simulink model "Microgrid_No_Attack"  (R2020b)
settings: Solver=VariableStepAuto  StartTime=0.0  StopTime=0.25  RelTol=1e-3
undefined symbols (not defined in the file): A_state_matrix_DG1, A_state_matrix_DG2, A_state_matrix_DG3, A_state_matrix_DG4, B_input_matrix_DG1, B_input_matrix_DG2, B_input_matrix_DG3, B_input_matrix_DG4, C_output_matrix_DG1, C_output_matrix_DG2, C_output_matrix_DG3, C_output_matrix_DG4, L_dot_DG1, L_dot_DG2, L_dot_DG3, L_dot_DG4
(part 2 of 2)

== matlab function Microgrid_No_Attack/vomag ==
  data: x9 input; x10 input; x24 input; vomag_1DG output; x25 input; x39 input; vomag_2DG output; vomag_3DG output; vomag_4DG output; x40 input; x54 input; x55 input
function [vomag_1DG,vomag_2DG,vomag_3DG,vomag_4DG] = vomag(x9,x10,x24,x25,x39,x40,x54,x55)


vomag_1DG= sqrt((x9^2) + (x10^2));
vomag_2DG= sqrt((x24^2) + (x25^2));
vomag_3DG= sqrt((x39^2) + (x40^2));
vomag_4DG= sqrt((x54^2) + (x55^2));

== matlab function Microgrid_No_Attack/NET ==
  data: x53 input; x54 input; x55 input; xdot53 output; xdot54 output; xdot55 output; xdot56 output; x56 input; x57 input; x58 input; vbD1 input; vbQ1 input; vbD2 input; vbQ2 input; vbD3 input; vbQ3 input; vbD4 input; vbQ4 input; xdot57 output; xdot58 output; wcom input
function [xdot53,xdot54,xdot55,xdot56,xdot57,xdot58] = Net(x53,x54,x55,x56,x57,x58,vbD1,vbQ1,vbD2,vbQ2,vbD3,vbQ3,vbD4,vbQ4,wcom)
% This block supports an embeddable subset of the MATLAB language.
% See the help menu for details. 
%%%--------Parameter values--------------
Cf=50e-6;Lf=1.35e-3;rLf=.1;
Lc=.35e-3;rLc=.03;
wc=31.41;
mp1=9.4e-5;mp2=mp1;mp3=12.5e-5;mp4=mp3;


nq1=1.3e-3;nq2=nq1;nq3=1.5e-3;nq4=nq3;


Kpv1=.1;Kiv1=420;Kpv2=Kpv1;Kiv2=Kiv1;
Kpc1=15;Kic1=20*10^3;Kpc2=Kpc1;Kic2=Kic1;


Kpv3=.05;Kiv3=390;Kpv4=Kpv3;Kiv4=Kiv3;
Kpc3=10.5;Kic3=16*10^3;Kpc4=Kpc3;Kic4=Kic3;


F=.75;

% kp=285;tau=0.00002;
%---------------
% rN=1e4;
% wb=2*pi*50;
% wref=2*pi*50;
% 
% Vn=380;
% Vdref=1*Vn;
% Vqref=0;
%-----Network Data-------
rline1=.23;Lline1=318e-6;
rline2=.35;Lline2=1847e-6;
rline3=.23;Lline3=318e-6;

Rload1=30;
Lload1=15/(2*pi*50);
Rload2=20;
Lload2=10/(2*pi*50);
Rload3=25;
Lload3=10/(2*pi*50);
Rload4=25;
Lload4=15/(2*pi*50);

%----1->2-----line1
xdot53=(-rline1/Lline1)*x53+wcom*x54+(1/Lline1)*(vbD1-vbD2); %ilineD1_dot
xdot54=(-rline1/Lline1)*x54-wcom*x53+(1/Lline1)*(vbQ1-vbQ2); %ilineQ1_dot
%----2->3-----line2
xdot55=(-rline2/Lline2)*x55+wcom*x56+(1/Lline2)*(vbD2-vbD3); %ilineD2_dot
xdot56=(-rline2/Lline2)*x56-wcom*x55+(1/Lline2)*(vbQ2-vbQ3); %ilineQ2_dot
%----3->4-----line3
xdot57=(-rline3/Lline3)*x57+wcom*x58+(1/Lline3)*(vbD3-vbD4); %ilineD3_dot
xdot58=(-rline3/Lline3)*x58-wcom*x57+(1/Lline3)*(vbQ3-vbQ4); %ilineQ3_dot

== matlab function Microgrid_No_Attack/LOAD ==
  data: x59 input; x60 input; x61 input; xdot59 output; xdot60 output; xdot61 output; xdot62 output; x62 input; x63 input; x64 input; x65 input; x66 input; vbD1 input; vbQ1 input; vbD2 input; vbQ2 input; vbD3 input; vbQ3 input; vbD4 input; vbQ4 input; wcom input; xdot63 output; xdot64 output; xdot65 output; xdot66 output
function [xdot59,xdot60,xdot61,xdot62,xdot63,xdot64,xdot65,xdot66] = Load(x59,x60,x61,x62,x63,x64,x65,x66,vbD1,vbQ1,vbD2,vbQ2,vbD3,vbQ3,vbD4,vbQ4,wcom)
% This block supports an embeddable subset of the MATLAB language.
% See the help menu for details. 
%%%--------Parameter values--------------
Cf=50e-6;Lf=1.35e-3;rLf=.1;
Lc=.35e-3;rLc=.03;
wc=31.41;
mp1=9.4e-5;mp2=mp1;mp3=12.5e-5;mp4=mp3;


nq1=1.3e-3;nq2=nq1;nq3=1.5e-3;nq4=nq3;


Kpv1=.1;Kiv1=420;Kpv2=Kpv1;Kiv2=Kiv1;
Kpc1=15;Kic1=20*10^3;Kpc2=Kpc1;Kic2=Kic1;


Kpv3=.05;Kiv3=390;Kpv4=Kpv3;Kiv4=Kiv3;
Kpc3=10.5;Kic3=16*10^3;Kpc4=Kpc3;Kic4=Kic3;


F=.75;

% kp=285;tau=0.00002;
%---------------
% rN=1e4;
% wb=2*pi*50;
% wref=2*pi*50;
% 
% Vn=380;
% Vdref=1*Vn;
% Vqref=0;
%-----Network Data-------
rline1=.23;Lline1=318e-6;
rline2=.35;Lline2=1847e-6;
rline3=.23;Lline3=318e-6;
% rline4=.35;Lline4=.58/(2*pi*50);
% rline5=.23;Lline5=.1/(2*pi*50);
% rline6=.35;Lline6=.58/(2*pi*50);
% rline7=.23;Lline7=.1/(2*pi*50);

Rload1=30;
Lload1=15/(2*pi*50);
Rload2=20;
Lload2=10/(2*pi*50);
Rload3=25;
Lload3=10/(2*pi*50);
Rload4=25;
Lload4=15/(2*pi*50);

%------Load1--------
xdot59=(-Rload1/Lload1)*x59+wcom*x60+(1/Lload1)*vbD1; %iloadD1_dot
xdot60=(-Rload1/Lload1)*x60-wcom*x59+(1/Lload1)*vbQ1; %iloadQ1_dot
%------Load2--------
xdot61=(-Rload2/Lload2)*x61+wcom*x62+(1/Lload2)*vbD2; %iloadD2_dot
xdot62=(-Rload2/Lload2)*x62-wcom*x61+(1/Lload2)*vbQ2; %iloadQ2_dot
%------Load3--------
xdot63=(-Rload3/Lload3)*x63+wcom*x64+(1/Lload3)*vbD3; %iloadD3_dot
xdot64=(-Rload3/Lload3)*x64-wcom*x63+(1/Lload3)*vbQ3; %iloadQ3_dot
%------Load4--------
xdot65=(-Rload4/Lload4)*x65+wcom*x66+(1/Lload4)*vbD4; %iloadD4_dot
xdot66=(-Rload4/Lload4)*x66-wcom*x65+(1/Lload4)*vbQ4; %iloadQ4_dot

== matlab function Microgrid_No_Attack/omega_1DG ==
  data: x1_1DG input; w1 output; x14_1DG input
function w1  = omega_1DG(x1_1DG,x14_1DG)

mp1=9.4e-5;mp2=mp1;mp3=12.5e-5;mp4=mp3;

w1= x14_1DG -mp1*x1_1DG;

== matlab function Microgrid_No_Attack/VB ==
  data: vbD1 output; vbQ1 output; vbD2 output; vbQ2 output; ilineD1 input; ilineQ1 input; ilineD2 input; vbD3 output; vbQ3 output; ilineQ2 input; ilineD3 input; ilineQ3 input; iloadD1 input; iloadQ1 input; iloadD2 input; iloadQ2 input; iloadD3 input; iloadQ3 input; iloadD4 input; iloadQ4 input; ioD1 input; ioQ1 input; ioD2 input; ioQ2 input; ioD3 input; ioQ3 input; ioD4 input; ioQ4 input; vbD4 output; vbQ4 output
function [vbD1,vbQ1,vbD2,vbQ2,vbD3,vbQ3,vbD4,vbQ4] = VB(ilineD1,ilineQ1,ilineD2,ilineQ2,ilineD3,ilineQ3,iloadD1,iloadQ1,iloadD2,iloadQ2,iloadD3,iloadQ3,iloadD4,iloadQ4,ioD1,ioQ1,ioD2,ioQ2,ioD3,ioQ3,ioD4,ioQ4)
% This block supports an embeddable subset of the MATLAB language.
% See the help menu for details. 
%%%--------Parameter values--------------


vbD1= (ioD1 - ilineD1 - iloadD1); vbQ1= (ioQ1 - ilineQ1 - iloadQ1);
vbD2= (ioD2 + ilineD1 - ilineD2 - iloadD2); vbQ2= (ioQ2 + ilineQ1 - ilineQ2 - iloadQ2);
vbD3= (ioD3 + ilineD2 - ilineD3 - iloadD3); vbQ3= (ioQ3 + ilineQ2 - ilineQ3 - iloadQ3);
vbD4= (ioD4 + ilineD3 - iloadD4); vbQ4= (ioQ4 + ilineQ3 - iloadQ4);

== matlab function Microgrid_No_Attack/omega_2DG ==
  data: x16_2DG input; w2 output; x29_2DG input
function w2  = omega_2DG(x16_2DG,x29_2DG)

mp1=9.4e-5;mp2=mp1;mp3=12.5e-5;mp4=mp3;

w2= x29_2DG -mp2*x16_2DG;

== matlab function Microgrid_No_Attack/omega_3DG ==
  data: x31_3DG input; w3 output; x44_3DG input
function w3  = omega_3DG(x31_3DG,x44_3DG)

mp1=9.4e-5;mp2=mp1;mp3=12.5e-5;mp4=mp3;

w3= x44_3DG -mp3*x31_3DG;

== matlab function Microgrid_No_Attack/Frequencies ==
  data: w1 input; f1 output; w2 input; w3 input; w4 input; f2 output; f3 output; f4 output
function [f1,f2,f3,f4] = frequencies(w1,w2,w3,w4)

f1 = w1/(2*pi);
f2 = w2/(2*pi);
f3 = w3/(2*pi);
f4 = w4/(2*pi);

== matlab function Microgrid_No_Attack/omega_4DG ==
  data: x46_4DG input; w4 output; x59_4DG input
function w4  = omega_4DG(x46_4DG,x59_4DG)

mp1=9.4e-5;mp2=mp1;mp3=12.5e-5;mp4=mp3;

w4= x59_4DG -mp4*x46_4DG;

== matlab function Microgrid_No_Attack/OBSERVER DG 1 ==
  data: A_state_matrix_DG1 input; x_hat_dot_DG1 output size=15; B_input_matrix_DG1 input; C_output_matrix_DG1 input; L_dot_DG1 input; y_DG1 input; u_vector_DG1 input; x1_hat input; x2_hat input; x3_hat input; x4_hat input; x5_hat input; x6_hat input; x7_hat input; x8_hat input; x9_hat input; x10_hat input; x11_hat input; x12_hat input; x13_hat input; x14_hat input; x15_hat input; y_hat_DG1 output size=15
function [x_hat_dot_DG1,y_hat_DG1] = observer_DG1(A_state_matrix_DG1,B_input_matrix_DG1,C_output_matrix_DG1,L_dot_DG1,y_DG1,u_vector_DG1, x1_hat,x2_hat,x3_hat,x4_hat,x5_hat,x6_hat,x7_hat,x8_hat,x9_hat,x10_hat,x11_hat,x12_hat,x13_hat,x14_hat,x15_hat)

Cf=50e-6;Lf=1.35e-3;rLf=.1;
Lc=.35e-3;rLc=.03;
wc=31.41;
mp1=9.4e-5;mp2=mp1;mp3=12.5e-5;mp4=mp3;


nq1=1.3e-3;nq2=nq1;nq3=1.5e-3;nq4=nq3;


Kpv1=.1;Kiv1=420;Kpv2=Kpv1;Kiv2=Kiv1;
Kpc1=15;Kic1=20*10^3;Kpc2=Kpc1;Kic2=Kic1;


Kpv3=.05;Kiv3=390;Kpv4=Kpv3;Kiv4=Kiv3;
Kpc3=10.5;Kic3=16*10^3;Kpc4=Kpc3;Kic4=Kic3;


F=.75;

wb=2*pi*50;

%% Non linear function (f) 15x1 

f_nonlinear_function_hat=[
(wc*x9_hat*x11_hat) + (wc*x10_hat*x12_hat);
(-wc*x9_hat*x12_hat) + (wc*x10_hat*x11_hat);
0;
0;
0;
0;
(x14_hat*x8_hat) - (mp1*x1_hat*x8_hat);
(-x14_hat*x7_hat) + (mp1*x1_hat*x7_hat);
(x14_hat*x10_hat) - (mp1*x1_hat*x10_hat);
(-x14_hat*x9_hat) + (mp1*x1_hat*x9_hat);
(x14_hat*x12_hat) - (mp1*x1_hat*x12_hat);
(-x14_hat*x11_hat) + (mp1*x1_hat*x11_hat);
0;
0;
0;
];

%% L'' hat DG 1

%L'' is 15x15, L' is 15x15, therefore L is 15x15

L_dot_dot_DG1= zeros(15,15)

L_dot_dot_DG1(1,7)= mp1*x8_hat;
L_dot_dot_DG1(1,8)= -mp1*x7_hat;
L_dot_dot_DG1(1,9)= mp1*x10_hat;
L_dot_dot_DG1(1,10)= -mp1*x9_hat;
L_dot_dot_DG1(1,11)= mp1*x12_hat - wc*x9_hat;
L_dot_dot_DG1(1,12)= -mp1*x11_hat - wc*x10_hat;
L_dot_dot_DG1(2,11)= -wc*x10_hat;
L_dot_dot_DG1(2,12)= wc*x9_hat;
L_dot_dot_DG1(7,14)= -x8_hat;
L_dot_dot_DG1(8,14)= x7_hat;
L_dot_dot_DG1(9,14)= -x10_hat;
L_dot_dot_DG1(10,14)= x9_hat;
L_dot_dot_DG1(11,14)= -x12_hat;
L_dot_dot_DG1(12,14)= x11_hat;



%% non linear gain L hat

L_hat_DG1= L_dot_DG1 + L_dot_dot_DG1

%% x hat vector

x_hat_vector_DG1= [x1_hat;x2_hat;x3_hat;x4_hat;x5_hat;x6_hat;x7_hat;x8_hat;x9_hat;x10_hat;x11_hat;x12_hat;x13_hat;x14_hat;x15_hat];
%% x hat dot

y_hat_DG1= C_output_matrix_DG1*x_hat_vector_DG1

x_hat_dot_DG1= A_state_matrix_DG1*x_hat_vector_DG1 + f_nonlinear_function_hat + B_input_matrix_DG1*u_vector_DG1 + L_hat_DG1*(y_DG1 - y_hat_DG1)

== matlab function Microgrid_No_Attack/DG 1 Matrices ==
  data: x1 input; x_dot_DG1 output; x2 input; x3 input; x4 input; x5 input; x6 input; x7 input; x8 input; x9 input; x10 input; x11 input; x12 input; x13 input; x14 input; x15 input; y_DG1 output; P_matrix input; Q_matrix input; w_matrix input; v_od_matrix input; wcom input; vbD1 input; vbQ1 input; A_state_matrix_DG1 input; B_input_matrix_DG1 input; C_output_matrix_DG1 input; ioD1 output; ioQ1 output; u_vector_DG1 output; vbd1 output; vbq1 output
function [x_dot_DG1, y_DG1, ioD1, ioQ1, u_vector_DG1,vbd1,vbq1] = Matrices_SSM_DG1(x1,x2,x3,x4,x5,x6,x7,x8,x9,x10,x11,x12,x13,x14,x15,P_matrix, Q_matrix, w_matrix, v_od_matrix,wcom,vbD1,vbQ1,A_state_matrix_DG1,B_input_matrix_DG1,C_output_matrix_DG1)



Cf=50e-6;Lf=1.35e-3;rLf=.1;
Lc=.35e-3;rLc=.03;
wc=31.41;
mp1=9.4e-5;mp2=mp1;mp3=12.5e-5;mp4=mp3;


nq1=1.3e-3;nq2=nq1;nq3=1.5e-3;nq4=nq3;


Kpv1=.1;Kiv1=420;Kpv2=Kpv1;Kiv2=Kiv1;
Kpc1=15;Kic1=20*10^3;Kpc2=Kpc1;Kic2=Kic1;


Kpv3=.05;Kiv3=390;Kpv4=Kpv3;Kiv4=Kiv3;
Kpc3=10.5;Kic3=16*10^3;Kpc4=Kpc3;Kic4=Kic3;


F=.75;

wb=2*pi*50;

A_matrix= [0 0 0 0; 1 0 0 0; 1 0 0 0; 1 0 0 0]; %associated adjacency matrix
g_pinning_gain= [1;0;0;0]; %pinning gain vector
w_ref= 2*pi*50;
v_ref= 1;
c_f_1DG= 30;
c_v_1DG= 30;

m_P_1DG= 9.4*10^-5;
m_P_2DG= 9.4*10^-5;
m_P_3DG= 12.5*10^-5;
m_P_4DG= 12.5*10^-5;
n_Q_1DG= 1.3*10^-3;
n_Q_2DG= 1.3*10^-3; 
n_Q_3DG= 1.5*10^-3; 
n_Q_4DG= 1.5*10^-3; 

m_P_matrix= [m_P_1DG; m_P_2DG; m_P_3DG; m_P_4DG];
n_Q_matrix= [n_Q_1DG; n_Q_2DG; n_Q_3DG; n_Q_4DG];

vbd1=cos(0)*vbD1+sin(0)*vbQ1;vbq1=-sin(0)*vbD1+cos(0)*vbQ1;

%% Extracting several terms for x dot 14

%Obtaining wj_input (cf*sum_aij*wj)

wj_input= 0;

for i=1
    for j= 1:4
        wj_input= (A_matrix(i,j)*w_matrix(j)) + wj_input;
    end
end

wj_input= wj_input*c_f_1DG;



%Obtaining wref_input (cf*gi*wref)


wref_input= c_f_1DG*g_pinning_gain(i)*w_ref;



%Obtaining Pj_input (cf*sum_aij*Pj)

Pj_input= 0;

for i= 1
    for j= 1:4
        Pj_input= (A_matrix(i,j)*m_P_matrix(j)*P_matrix(j)) + Pj_input;
    end
end

Pj_input= Pj_input*c_f_1DG;


        
%% Extracting several terms for x dot 15


%Obtaining vodj_input (cv*sum_aij*vodj)

vodj_input= 0;

for i= 1
    for j= 1:4
        vodj_input= (A_matrix(i,j)*v_od_matrix(j)) + vodj_input;
    end
end

vodj_input= c_v_1DG*vodj_input;


%Obtaining vref_input (cv*gi*vref)

vref_input= c_v_1DG*g_pinning_gain(i)*v_ref;


%Obtaining Qj_input (cv*sum_aij*Qj)

Qj_input= 0;

for i= 1
    for j= 1:4
        Qj_input= (A_matrix(i,j)*n_Q_matrix(j)*Q_matrix(j)) + Qj_input;
    end
end

Qj_input= c_v_1DG*Qj_input;




%% A matrix calculation

%A has 15 rows 15 columns

% x_vector=[P_i, Q_i, fi_d_i, fi_q_i,gamma_d_i,gamma_q_i, il_d_i, il_q_i, vo_d_i, vo_q_i,io_d_i,io_q_i,alpha_i,wni,Vni];


%% B Matrix Calculation 

%B has 15 rows 9 columns

u_vector_DG1= [wcom;vbd1;vbq1;wj_input;wref_input;Pj_input;vodj_input;vref_input;Qj_input];



%% C matrix calculation

% y=[states from 1 to 15]

%C has 15 rows 15 columns, C equal to identity matrix


%% Non linear function (f) 15x1 

f_nonlinear_function=[
(wc*x9*x11) + (wc*x10*x12);
(-wc*x9*x12) + (wc*x10*x11);
0;
0;
0;
0;
(x14*x8) - (mp1*x1*x8);
(-x14*x7) + (mp1*x1*x7);
(x14*x10) - (mp1*x1*x10);
(-x14*x9) + (mp1*x1*x9);
(x14*x12) - (mp1*x1*x12);
(-x14*x11) + (mp1*x1*x11);
0;
0;
0;
];


%% x vector

x_vector_DG1= [x1;x2;x3;x4;x5;x6;x7;x8;x9;x10;x11;x12;x13;x14;x15];
%% xdot
x_dot_DG1= A_state_matrix_DG1*x_vector_DG1 + f_nonlinear_function + B_input_matrix_DG1*u_vector_DG1

y_DG1= C_output_matrix_DG1*x_vector_DG1



ioD1=cos(0)*x11-sin(0)*x12;
ioQ1=sin(0)*x11+cos(0)*x12;

== matlab function Microgrid_No_Attack/OBSERVER DG 2 ==
  data: A_state_matrix_DG2 input; x_hat_dot_DG2 output; B_input_matrix_DG2 input; C_output_matrix_DG2 input; L_dot_DG2 input; y_DG2 input; u_vector_DG2 input; x1_hat input; x2_hat input; x3_hat input; x4_hat input; x5_hat input; x6_hat input; x7_hat input; x8_hat input; x9_hat input; x10_hat input; x11_hat input; x12_hat input; x13_hat input; x14_hat input; x15_hat input; y_hat_DG2 output
function [x_hat_dot_DG2,y_hat_DG2] = observer_DG2(A_state_matrix_DG2,B_input_matrix_DG2,C_output_matrix_DG2,L_dot_DG2,y_DG2,u_vector_DG2, x1_hat,x2_hat,x3_hat,x4_hat,x5_hat,x6_hat,x7_hat,x8_hat,x9_hat,x10_hat,x11_hat,x12_hat,x13_hat,x14_hat,x15_hat)

Cf=50e-6;Lf=1.35e-3;rLf=.1;
Lc=.35e-3;rLc=.03;
wc=31.41;
mp1=9.4e-5;mp2=mp1;mp3=12.5e-5;mp4=mp3;


nq1=1.3e-3;nq2=nq1;nq3=1.5e-3;nq4=nq3;


Kpv1=.1;Kiv1=420;Kpv2=Kpv1;Kiv2=Kiv1;
Kpc1=15;Kic1=20*10^3;Kpc2=Kpc1;Kic2=Kic1;


Kpv3=.05;Kiv3=390;Kpv4=Kpv3;Kiv4=Kiv3;
Kpc3=10.5;Kic3=16*10^3;Kpc4=Kpc3;Kic4=Kic3;


F=.75;

wb=2*pi*50;

%% Non linear function (f) 15x1 

f_nonlinear_function_hat=[
(wc*x9_hat*x11_hat) + (wc*x10_hat*x12_hat);
(-wc*x9_hat*x12_hat) + (wc*x10_hat*x11_hat);
0;
0;
0;
0;
(x14_hat*x8_hat) - (mp1*x1_hat*x8_hat);
(-x14_hat*x7_hat) + (mp1*x1_hat*x7_hat);
(x14_hat*x10_hat) - (mp1*x1_hat*x10_hat);
(-x14_hat*x9_hat) + (mp1*x1_hat*x9_hat);
(x14_hat*x12_hat) - (mp1*x1_hat*x12_hat);
(-x14_hat*x11_hat) + (mp1*x1_hat*x11_hat);
0;
0;
0;
];

%% L'' hat DG 2

%L'' is 15x15, L' is 15x15, therefore L is 15x15

L_dot_dot_DG2= zeros(15,15)

L_dot_dot_DG2(1,7)= mp2*x8_hat;
L_dot_dot_DG2(1,8)= -mp2*x7_hat;
L_dot_dot_DG2(1,9)= mp2*x10_hat;
L_dot_dot_DG2(1,10)= -mp2*x9_hat;
L_dot_dot_DG2(1,11)= mp2*x12_hat - wc*x9_hat;
L_dot_dot_DG2(1,12)= -mp2*x11_hat - wc*x10_hat;
L_dot_dot_DG2(2,11)= -wc*x10_hat;
L_dot_dot_DG2(2,12)= wc*x9_hat;
L_dot_dot_DG2(7,14)= -x8_hat;
L_dot_dot_DG2(8,14)= x7_hat;
L_dot_dot_DG2(9,14)= -x10_hat;
L_dot_dot_DG2(10,14)= x9_hat;
L_dot_dot_DG2(11,14)= -x12_hat;
L_dot_dot_DG2(12,14)= x11_hat;

%% non linear gain L hat

L_hat_DG2= L_dot_DG2 + L_dot_dot_DG2

%% x hat vector

x_hat_vector_DG2= [x1_hat;x2_hat;x3_hat;x4_hat;x5_hat;x6_hat;x7_hat;x8_hat;x9_hat;x10_hat;x11_hat;x12_hat;x13_hat;x14_hat;x15_hat];
%% x hat dot

y_hat_DG2= C_output_matrix_DG2*x_hat_vector_DG2

x_hat_dot_DG2= A_state_matrix_DG2*x_hat_vector_DG2 + f_nonlinear_function_hat + B_input_matrix_DG2*u_vector_DG2 + L_hat_DG2*(y_DG2 - y_hat_DG2)

== matlab function Microgrid_No_Attack/OBSERVER DG 3 ==
  data: A_state_matrix_DG3 input; x_hat_dot_DG3 output; B_input_matrix_DG3 input; C_output_matrix_DG3 input; L_dot_DG3 input; y_DG3 input; u_vector_DG3 input; x1_hat input; x2_hat input; x3_hat input; x4_hat input; x5_hat input; x6_hat input; x7_hat input; x8_hat input; x9_hat input; x10_hat input; x11_hat input; x12_hat input; x13_hat input; x14_hat input; x15_hat input; y_hat_DG3 output
function [x_hat_dot_DG3,y_hat_DG3] = observer_DG3(A_state_matrix_DG3,B_input_matrix_DG3,C_output_matrix_DG3,L_dot_DG3,y_DG3,u_vector_DG3, x1_hat,x2_hat,x3_hat,x4_hat,x5_hat,x6_hat,x7_hat,x8_hat,x9_hat,x10_hat,x11_hat,x12_hat,x13_hat,x14_hat,x15_hat)

Cf=50e-6;Lf=1.35e-3;rLf=.1;
Lc=.35e-3;rLc=.03;
wc=31.41;
mp1=9.4e-5;mp2=mp1;mp3=12.5e-5;mp4=mp3;


nq1=1.3e-3;nq2=nq1;nq3=1.5e-3;nq4=nq3;


Kpv1=.1;Kiv1=420;Kpv2=Kpv1;Kiv2=Kiv1;
Kpc1=15;Kic1=20*10^3;Kpc2=Kpc1;Kic2=Kic1;


Kpv3=.05;Kiv3=390;Kpv4=Kpv3;Kiv4=Kiv3;
Kpc3=10.5;Kic3=16*10^3;Kpc4=Kpc3;Kic4=Kic3;


F=.75;

wb=2*pi*50;

%% Non linear function (f) 15x1 

f_nonlinear_function_hat=[
(wc*x9_hat*x11_hat) + (wc*x10_hat*x12_hat);
(-wc*x9_hat*x12_hat) + (wc*x10_hat*x11_hat);
0;
0;
0;
0;
(x14_hat*x8_hat) - (mp3*x1_hat*x8_hat);
(-x14_hat*x7_hat) + (mp3*x1_hat*x7_hat);
(x14_hat*x10_hat) - (mp3*x1_hat*x10_hat);
(-x14_hat*x9_hat) + (mp3*x1_hat*x9_hat);
(x14_hat*x12_hat) - (mp3*x1_hat*x12_hat);
(-x14_hat*x11_hat) + (mp3*x1_hat*x11_hat);
0;
0;
0;
];

%% L'' hat DG 3

%L'' is 15x15, L' is 15x15, therefore L is 15x15

L_dot_dot_DG3= zeros(15,15)

L_dot_dot_DG3(1,7)= mp3*x8_hat;
L_dot_dot_DG3(1,8)= -mp3*x7_hat;
L_dot_dot_DG3(1,9)= mp3*x10_hat;
L_dot_dot_DG3(1,10)= -mp3*x9_hat;
L_dot_dot_DG3(1,11)= mp3*x12_hat - wc*x9_hat;
L_dot_dot_DG3(1,12)= -mp3*x11_hat - wc*x10_hat;
L_dot_dot_DG3(2,11)= -wc*x10_hat;
L_dot_dot_DG3(2,12)= wc*x9_hat;
L_dot_dot_DG3(7,14)= -x8_hat;
L_dot_dot_DG3(8,14)= x7_hat;
L_dot_dot_DG3(9,14)= -x10_hat;
L_dot_dot_DG3(10,14)= x9_hat;
L_dot_dot_DG3(11,14)= -x12_hat;
L_dot_dot_DG3(12,14)= x11_hat;

%% non linear gain L hat

L_hat_DG3= L_dot_DG3 + L_dot_dot_DG3

%% x hat vector

x_hat_vector_DG3= [x1_hat;x2_hat;x3_hat;x4_hat;x5_hat;x6_hat;x7_hat;x8_hat;x9_hat;x10_hat;x11_hat;x12_hat;x13_hat;x14_hat;x15_hat];
%% x hat dot

y_hat_DG3= C_output_matrix_DG3*x_hat_vector_DG3

x_hat_dot_DG3= A_state_matrix_DG3*x_hat_vector_DG3 + f_nonlinear_function_hat + B_input_matrix_DG3*u_vector_DG3 + L_hat_DG3*(y_DG3 - y_hat_DG3)

== matlab function Microgrid_No_Attack/OBSERVER DG 4 ==
  data: A_state_matrix_DG4 input; x_hat_dot_DG4 output size=15; B_input_matrix_DG4 input; C_output_matrix_DG4 input; L_dot_DG4 input; y_DG4 input; u_vector_DG4 input; x1_hat input; x2_hat input; x3_hat input; x4_hat input; x5_hat input; x6_hat input; x7_hat input; x8_hat input; x9_hat input; x10_hat input; x11_hat input; x12_hat input; x13_hat input; x14_hat input; x15_hat input; y_hat_DG4 output size=15
function [x_hat_dot_DG4,y_hat_DG4] = observer_DG4(A_state_matrix_DG4,B_input_matrix_DG4,C_output_matrix_DG4,L_dot_DG4,y_DG4,u_vector_DG4, x1_hat,x2_hat,x3_hat,x4_hat,x5_hat,x6_hat,x7_hat,x8_hat,x9_hat,x10_hat,x11_hat,x12_hat,x13_hat,x14_hat,x15_hat)

Cf=50e-6;Lf=1.35e-3;rLf=.1;
Lc=.35e-3;rLc=.03;
wc=31.41;
mp1=9.4e-5;mp2=mp1;mp3=12.5e-5;mp4=mp3;


nq1=1.3e-3;nq2=nq1;nq3=1.5e-3;nq4=nq3;


Kpv1=.1;Kiv1=420;Kpv2=Kpv1;Kiv2=Kiv1;
Kpc1=15;Kic1=20*10^3;Kpc2=Kpc1;Kic2=Kic1;


Kpv3=.05;Kiv3=390;Kpv4=Kpv3;Kiv4=Kiv3;
Kpc3=10.5;Kic3=16*10^3;Kpc4=Kpc3;Kic4=Kic3;


F=.75;

wb=2*pi*50;

%% Non linear function (f) 15x1 

f_nonlinear_function_hat=[
(wc*x9_hat*x11_hat) + (wc*x10_hat*x12_hat);
(-wc*x9_hat*x12_hat) + (wc*x10_hat*x11_hat);
0;
0;
0;
0;
(x14_hat*x8_hat) - (mp3*x1_hat*x8_hat);
(-x14_hat*x7_hat) + (mp3*x1_hat*x7_hat);
(x14_hat*x10_hat) - (mp3*x1_hat*x10_hat);
(-x14_hat*x9_hat) + (mp3*x1_hat*x9_hat);
(x14_hat*x12_hat) - (mp3*x1_hat*x12_hat);
(-x14_hat*x11_hat) + (mp3*x1_hat*x11_hat);
0;
0;
0;
];

%% L'' hat DG 4

%L'' is 15x15, L' is 15x15, therefore L is 15x15

L_dot_dot_DG4= zeros(15,15)

L_dot_dot_DG4(1,7)= mp4*x8_hat;
L_dot_dot_DG4(1,8)= -mp4*x7_hat;
L_dot_dot_DG4(1,9)= mp4*x10_hat;
L_dot_dot_DG4(1,10)= -mp4*x9_hat;
L_dot_dot_DG4(1,11)= mp4*x12_hat - wc*x9_hat;
L_dot_dot_DG4(1,12)= -mp4*x11_hat - wc*x10_hat;
L_dot_dot_DG4(2,11)= -wc*x10_hat;
L_dot_dot_DG4(2,12)= wc*x9_hat;
L_dot_dot_DG4(7,14)= -x8_hat;
L_dot_dot_DG4(8,14)= x7_hat;
L_dot_dot_DG4(9,14)= -x10_hat;
L_dot_dot_DG4(10,14)= x9_hat;
L_dot_dot_DG4(11,14)= -x12_hat;
L_dot_dot_DG4(12,14)= x11_hat;


%% non linear gain L hat

L_hat_DG4= L_dot_DG4 + L_dot_dot_DG4

%% x hat vector

x_hat_vector_DG4= [x1_hat;x2_hat;x3_hat;x4_hat;x5_hat;x6_hat;x7_hat;x8_hat;x9_hat;x10_hat;x11_hat;x12_hat;x13_hat;x14_hat;x15_hat];
%% x hat dot

y_hat_DG4= C_output_matrix_DG4*x_hat_vector_DG4

x_hat_dot_DG4= A_state_matrix_DG4*x_hat_vector_DG4 + f_nonlinear_function_hat + B_input_matrix_DG4*u_vector_DG4 + L_hat_DG4*(y_DG4 - y_hat_DG4)

== matlab function Microgrid_No_Attack/omega_1DG_observer ==
  data: x1_hat_1DG input; w1_observer output; x14_hat_1DG input
function w1_observer  = omega_1DG_observer(x1_hat_1DG,x14_hat_1DG)

mp1=9.4e-5;mp2=mp1;mp3=12.5e-5;mp4=mp3;

w1_observer= x14_hat_1DG -mp1*x1_hat_1DG;

== matlab function Microgrid_No_Attack/Frequencies1 ==
  data: w1 input; f1 output; w2 input; w3 input; w4 input; f2 output; f3 output; f4 output
function [f1,f2,f3,f4] = frequencies(w1,w2,w3,w4)

f1 = w1/(2*pi);
f2 = w2/(2*pi);
f3 = w3/(2*pi);
f4 = w4/(2*pi);

== matlab function Microgrid_No_Attack/vomag1 ==
  data: x9 input; x10 input; x24 input; vomag_1DG output; x25 input; x39 input; vomag_2DG output; vomag_3DG output; vomag_4DG output; x40 input; x54 input; x55 input
function [vomag_1DG,vomag_2DG,vomag_3DG,vomag_4DG] = vomag(x9,x10,x24,x25,x39,x40,x54,x55)


vomag_1DG= sqrt((x9^2) + (x10^2));
vomag_2DG= sqrt((x24^2) + (x25^2));
vomag_3DG= sqrt((x39^2) + (x40^2));
vomag_4DG= sqrt((x54^2) + (x55^2));

== matlab function Microgrid_No_Attack/omega_2DG_observer ==
  data: x16_hat_2DG input; w2_observer output; x29_hat_2DG input
function w2_observer  = omega_2DG_observer(x16_hat_2DG,x29_hat_2DG)

mp1=9.4e-5;mp2=mp1;mp3=12.5e-5;mp4=mp3;

w2_observer= x29_hat_2DG -mp2*x16_hat_2DG;

== matlab function Microgrid_No_Attack/omega_3DG_observer ==
  data: x31_hat_3DG input; w3_observer output; x44_hat_3DG input
function w3_observer  = omega_3DG_observer(x31_hat_3DG,x44_hat_3DG)

mp1=9.4e-5;mp2=mp1;mp3=12.5e-5;mp4=mp3;

w3_observer= x44_hat_3DG -mp3*x31_hat_3DG;

== matlab function Microgrid_No_Attack/omega_4DG_observer ==
  data: x46_hat_4DG input; w4_observer output; x59_hat_4DG input
function w4_observer  = omega_4DG_observer(x46_hat_4DG,x59_hat_4DG)

mp1=9.4e-5;mp2=mp1;mp3=12.5e-5;mp4=mp3;

w4_observer= x59_hat_4DG -mp4*x46_hat_4DG;

== matlab function Microgrid_No_Attack/MATLAB Function1 ==
  data: x_vector_DG1 input; L1_DG1 output; x_vector_DG4 input; x_hat_vector_DG1 input; x_hat_vector_DG4 input; L2_DG1 output; L1_DG4 output; L2_DG4 output
function [L1_DG1, L2_DG1, L1_DG4, L2_DG4] = norm_residual_error(x_vector_DG1,x_vector_DG4,x_hat_vector_DG1,x_hat_vector_DG4)

L1_DG1= norm(x_vector_DG1-x_hat_vector_DG1,1);
L2_DG1= norm(x_vector_DG1-x_hat_vector_DG1,2);
L1_DG4= norm(x_vector_DG4-x_hat_vector_DG4,1);
L2_DG4= norm(x_vector_DG4-x_hat_vector_DG4,2);

== matlab function Microgrid_No_Attack/DG 2 Matrices ==
  data: x1 input; x_dot_DG2 output; x2 input; x3 input; x4 input; x5 input; x6 input; x7 input; x8 input; x9 input; x10 input; x11 input; x12 input; x13 input; x14 input; x15 input; y_DG2 output; P_matrix input; Q_matrix input; w_matrix input; v_od_matrix input; wcom input; vbD2 input; vbQ2 input; A_state_matrix_DG2 input; B_input_matrix_DG2 input; C_output_matrix_DG2 input; ioD2 output; ioQ2 output; u_vector_DG2 output; vbd2 output; vbq2 output
function [x_dot_DG2, y_DG2,ioD2,ioQ2, u_vector_DG2,vbd2,vbq2] = Matrices_SSM_DG2(x1,x2,x3,x4,x5,x6,x7,x8,x9,x10,x11,x12,x13,x14,x15,P_matrix, Q_matrix, w_matrix, v_od_matrix,wcom,vbD2,vbQ2,A_state_matrix_DG2,B_input_matrix_DG2,C_output_matrix_DG2)



Cf=50e-6;Lf=1.35e-3;rLf=.1;
Lc=.35e-3;rLc=.03;
wc=31.41;
mp1=9.4e-5;mp2=mp1;mp3=12.5e-5;mp4=mp3;


nq1=1.3e-3;nq2=nq1;nq3=1.5e-3;nq4=nq3;


Kpv1=.1;Kiv1=420;Kpv2=Kpv1;Kiv2=Kiv1;
Kpc1=15;Kic1=20*10^3;Kpc2=Kpc1;Kic2=Kic1;


Kpv3=.05;Kiv3=390;Kpv4=Kpv3;Kiv4=Kiv3;
Kpc3=10.5;Kic3=16*10^3;Kpc4=Kpc3;Kic4=Kic3;


F=.75;

wb=2*pi*50;

A_matrix= [0 0 0 0; 1 0 0 0; 1 0 0 0; 1 0 0 0]; %associated adjacency matrix
g_pinning_gain= [1;0;0;0]; %pinning gain vector
w_ref= 2*pi*50;
v_ref= 1;
c_f_2DG= 30;
c_v_2DG= 30;

m_P_1DG= 9.4*10^-5;
m_P_2DG= 9.4*10^-5;
m_P_3DG= 12.5*10^-5;
m_P_4DG= 12.5*10^-5;
n_Q_1DG= 1.3*10^-3;
n_Q_2DG= 1.3*10^-3; 
n_Q_3DG= 1.5*10^-3; 
n_Q_4DG= 1.5*10^-3; 

m_P_matrix= [m_P_1DG; m_P_2DG; m_P_3DG; m_P_4DG];
n_Q_matrix= [n_Q_1DG; n_Q_2DG; n_Q_3DG; n_Q_4DG];

vbd2=cos(x13)*vbD2+sin(x13)*vbQ2;vbq2=-sin(x13)*vbD2+cos(x13)*vbQ2;



%% Extracting several terms for x dot 14



%Obtaining wj_input (cf*sum_aij*wj)

wj_input= 0;

for i=2
    for j= 1:4
        wj_input= (A_matrix(i,j)*w_matrix(j)) + wj_input;
    end
end

wj_input= wj_input*c_f_2DG;



%Obtaining wref_input (cf*gi*wref)


wref_input= c_f_2DG*g_pinning_gain(i)*w_ref;



%Obtaining Pj_input (cf*sum_aij*Pj)

Pj_input= 0;

for i= 2
    for j= 1:4
        Pj_input= (A_matrix(i,j)*m_P_matrix(j)*P_matrix(j)) + Pj_input;
    end
end

Pj_input= Pj_input*c_f_2DG;


        
%% Extracting several terms for x dot 15



%Obtaining vodj_input (cv*sum_aij*vodj)

vodj_input= 0;

for i= 2
    for j= 1:4
        vodj_input= (A_matrix(i,j)*v_od_matrix(j)) + vodj_input;
    end
end

vodj_input= c_v_2DG*vodj_input;


%Obtaining vref_input (cv*gi*vref)

vref_input= c_v_2DG*g_pinning_gain(i)*v_ref;


%Obtaining Qj_input (cv*sum_aij*Qj)

Qj_input= 0;

for i= 2
    for j= 1:4
        Qj_input= (A_matrix(i,j)*n_Q_matrix(j)*Q_matrix(j)) + Qj_input;
    end
end

Qj_input= c_v_2DG*Qj_input;




%% A matrix calculation

%A has 15 rows 15 columns

% x_vector=[alpha_i, P_i, Q_i, fi_d_i, fi_q_i,gamma_d_i,gamma_q_i, il_d_i, il_q_i, vo_d_i, vo_q_i,io_d_i,io_q_i,wni,Vni];


%% B Matrix Calculation 

%B has 15 rows 9 columns

u_vector_DG2= [wcom;vbd2;vbq2;wj_input;wref_input;Pj_input;vodj_input;vref_input;Qj_input];


%% C matrix calculation

% y=[wi; vodi; Pi; Qi;]

%C has 4 rows 15 columns


%% Non linear function (f) 15x1 

f_nonlinear_function=[
(wc*x9*x11) + (wc*x10*x12);
(-wc*x9*x12) + (wc*x10*x11);
0;
0;
0;
0;
(x14*x8) - (mp1*x1*x8);
(-x14*x7) + (mp1*x1*x7);
(x14*x10) - (mp1*x1*x10);
(-x14*x9) + (mp1*x1*x9);
(x14*x12) - (mp1*x1*x12);
(-x14*x11) + (mp1*x1*x11);
0;
0;
0;
];



%% x vector

x_vector_DG2= [x1;x2;x3;x4;x5;x6;x7;x8;x9;x10;x11;x12;x13;x14;x15];
%% xdot
x_dot_DG2= A_state_matrix_DG2*x_vector_DG2 + f_nonlinear_function + B_input_matrix_DG2*u_vector_DG2

y_DG2= C_output_matrix_DG2*x_vector_DG2


ioD2=cos(x13)*x11-sin(x13)*x12;
ioQ2=sin(x13)*x11+cos(x13)*x12;

== matlab function Microgrid_No_Attack/DG 3 Matrices ==
  data: x1 input; x_dot_DG3 output; x2 input; x3 input; x4 input; x5 input; x6 input; x7 input; x8 input; x9 input; x10 input; x11 input; x12 input; x13 input; x14 input; x15 input; y_DG3 output; P_matrix input; Q_matrix input; w_matrix input; v_od_matrix input; wcom input; vbD3 input; vbQ3 input; A_state_matrix_DG3 input; B_input_matrix_DG3 input; C_output_matrix_DG3 input; ioD3 output; ioQ3 output; u_vector_DG3 output; vbd3 output; vbq3 output
function [x_dot_DG3, y_DG3,ioD3,ioQ3,u_vector_DG3,vbd3,vbq3] = Matrices_SSM_DG3(x1,x2,x3,x4,x5,x6,x7,x8,x9,x10,x11,x12,x13,x14,x15,P_matrix, Q_matrix, w_matrix, v_od_matrix,wcom,vbD3,vbQ3,A_state_matrix_DG3,B_input_matrix_DG3,C_output_matrix_DG3)



Cf=50e-6;Lf=1.35e-3;rLf=.1;
Lc=.35e-3;rLc=.03;
wc=31.41;
mp1=9.4e-5;mp2=mp1;mp3=12.5e-5;mp4=mp3;


nq1=1.3e-3;nq2=nq1;nq3=1.5e-3;nq4=nq3;


Kpv1=.1;Kiv1=420;Kpv2=Kpv1;Kiv2=Kiv1;
Kpc1=15;Kic1=20*10^3;Kpc2=Kpc1;Kic2=Kic1;


Kpv3=.05;Kiv3=390;Kpv4=Kpv3;Kiv4=Kiv3;
Kpc3=10.5;Kic3=16*10^3;Kpc4=Kpc3;Kic4=Kic3;


F=.75;

wb=2*pi*50;

A_matrix= [0 0 0 0; 1 0 0 0; 1 0 0 0; 1 0 0 0]; %associated adjacency matrix
g_pinning_gain= [1;0;0;0]; %pinning gain vector
w_ref= 2*pi*50;
v_ref= 1;
c_f_2DG= 30;
c_v_2DG= 30;

m_P_1DG= 9.4*10^-5;
m_P_2DG= 9.4*10^-5;
m_P_3DG= 12.5*10^-5;
m_P_4DG= 12.5*10^-5;
n_Q_1DG= 1.3*10^-3;
n_Q_2DG= 1.3*10^-3; 
n_Q_3DG= 1.5*10^-3; 
n_Q_4DG= 1.5*10^-3; 

m_P_matrix= [m_P_1DG; m_P_2DG; m_P_3DG; m_P_4DG];
n_Q_matrix= [n_Q_1DG; n_Q_2DG; n_Q_3DG; n_Q_4DG];

vbd3=cos(x13)*vbD3+sin(x13)*vbQ3;vbq3=-sin(x13)*vbD3+cos(x13)*vbQ3;



%% Extracting several terms for x dot 14



%Obtaining wj_input (cf*sum_aij*wj)

wj_input= 0;

for i=3
    for j= 1:4
        wj_input= (A_matrix(i,j)*w_matrix(j)) + wj_input;
    end
end

wj_input= wj_input*c_f_2DG;



%Obtaining wref_input (cf*gi*wref)


wref_input= c_f_2DG*g_pinning_gain(i)*w_ref;



%Obtaining Pj_input (cf*sum_aij*Pj)

Pj_input= 0;

for i= 3
    for j= 1:4
        Pj_input= (A_matrix(i,j)*m_P_matrix(j)*P_matrix(j)) + Pj_input;
    end
end

Pj_input= Pj_input*c_f_2DG;


        
%% Extracting several terms for x dot 15



%Obtaining vodj_input (cv*sum_aij*vodj)

vodj_input= 0;

for i= 3
    for j= 1:4
        vodj_input= (A_matrix(i,j)*v_od_matrix(j)) + vodj_input;
    end
end

vodj_input= c_v_2DG*vodj_input;


%Obtaining vref_input (cv*gi*vref)

vref_input= c_v_2DG*g_pinning_gain(i)*v_ref;


%Obtaining Qj_input (cv*sum_aij*Qj)

Qj_input= 0;

for i= 3
    for j= 1:4
        Qj_input= (A_matrix(i,j)*n_Q_matrix(j)*Q_matrix(j)) + Qj_input;
    end
end

Qj_input= c_v_2DG*Qj_input;




%% A matrix calculation

%A has 15 rows 15 columns

% x_vector=[alpha_i, P_i, Q_i, fi_d_i, fi_q_i,gamma_d_i,gamma_q_i, il_d_i, il_q_i, vo_d_i, vo_q_i,io_d_i,io_q_i,wni,Vni];


%% B Matrix Calculation 

%B has 15 rows 9 columns

u_vector_DG3= [wcom;vbd3;vbq3;wj_input;wref_input;Pj_input;vodj_input;vref_input;Qj_input];



%% C matrix calculation

% y=[wi; vodi; Pi; Qi;]

%C has 4 rows 15 columns



%% Non linear function (f) 15x1 

f_nonlinear_function=[
(wc*x9*x11) + (wc*x10*x12);
(-wc*x9*x12) + (wc*x10*x11);
0;
0;
0;
0;
(x14*x8) - (mp3*x1*x8);
(-x14*x7) + (mp3*x1*x7);
(x14*x10) - (mp3*x1*x10);
(-x14*x9) + (mp3*x1*x9);
(x14*x12) - (mp3*x1*x12);
(-x14*x11) + (mp3*x1*x11);
0;
0;
0;
];



%% x vector

x_vector_DG3= [x1;x2;x3;x4;x5;x6;x7;x8;x9;x10;x11;x12;x13;x14;x15];
%% xdot
x_dot_DG3= A_state_matrix_DG3*x_vector_DG3 + f_nonlinear_function + B_input_matrix_DG3*u_vector_DG3

y_DG3= C_output_matrix_DG3*x_vector_DG3


ioD3=cos(x13)*x11-sin(x13)*x12;
ioQ3=sin(x13)*x11+cos(x13)*x12;
